simulink model "Chua_TxRx"  (R2020a)
settings: Solver=VariableStepAuto  StartTime=0.0  StopTime=140  RelTol=1e-3
values from neighbouring files (symbols this model uses):
  beta = -36    [SetupConstants.m]
  delay = 10    [SetupConstants.m]
  freq = 1/10    (= 0.1)    [SetupConstants.m]
libraries: simulink x1
settings Model: PacingRate=1.100000  Creator=RaviM  LastModifiedBy=RaviM

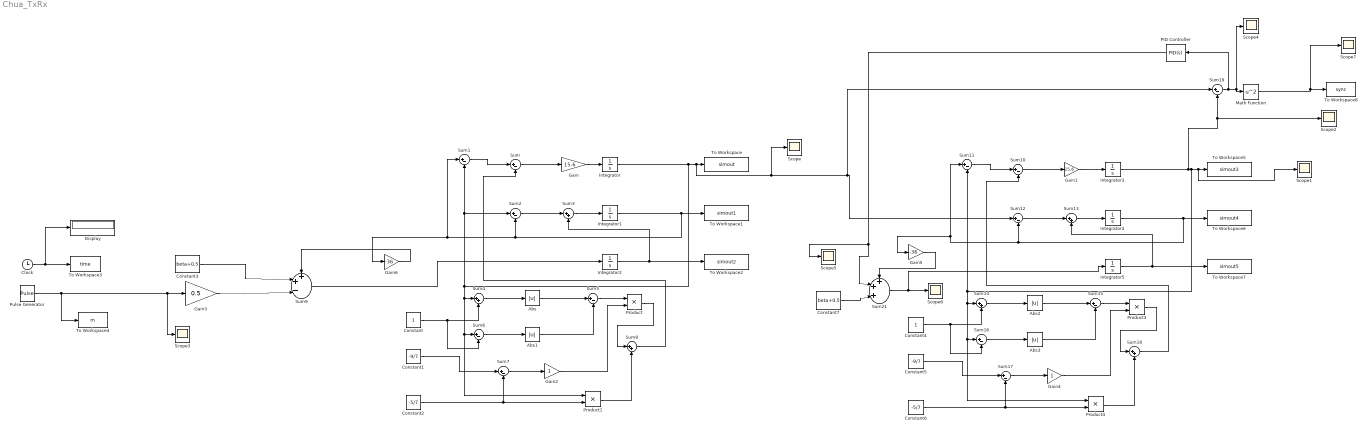
== system Chua_TxRx ==
  Abs{,1..3} (4 alike) : Abs
  Clock : Clock
  Constant : Constant
  Constant1 : Constant  Value=-9/7
  Constant2 : Constant  Value=-5/7
  Constant3 : Constant  Value=beta+0.5
  Constant4 : Constant
  Constant5 : Constant  Value=-9/7
  Constant6 : Constant  Value=-5/7
  Constant7 : Constant  Value=beta+0.5
  Display : Display
      settings: Decimation=5
  Gain : Gain  Gain=15.6
  Gain1 : Gain  Gain=15.6
  Gain2 : Gain
  Gain3 : Gain  Gain=0.5
  Gain4 : Gain
  Gain5 : Gain  Gain=-36
  Gain6 : Gain  Gain=-36
  Integrator{,1..5} (6 alike) : Integrator  InitialCondition=0.1
  Math Function : Math  Operator=square  SignedPower=on  SaturateOnIntegerOverflow=on
  PID Controller : simulink/Continuous/PID Controller  Controller=PID  Form=Ideal  TimeDomain=Continuous-time  UseExternalTs=off  SampleTime=-1  IntegratorMethod=Forward Euler  FilterMethod=Forward Euler  ControllerParametersSource=internal  P=.5  I=0.2  D=.0000004  UseFilter=on  N=100  TunerSelectOption=Transfer Function Based (PID Tuner App)  InitialConditionSource=internal  InitialConditionForIntegrator=0  InitialConditionForFilter=0  DifferentiatorICPrevScaledInput=0  ExternalReset=none  TrackingMode=off  Kt=1  LimitOutput=off  UpperSaturationLimit=inf  LowerSaturationLimit=-inf  LinearizeAsGain=on  AntiWindupMode=none  Kb=1  POutMin=[]  POutMax=[]  IOutMin=[]  IOutMax=[]  DOutMin=[]  DOutMax=[]  NOutMin=[]  NOutMax=[]  SumOutMin=[]  SumOutMax=[]  SaturationOutMin=[]  SaturationOutMax=[]  PParamMin=[]  PParamMax=[]  IParamMin=[]  IParamMax=[]  DParamMin=[]  DParamMax=[]  NParamMin=[]  NParamMax=[]  KbParamMin=[]  KbParamMax=[]  KtParamMin=[]  KtParamMax=[]  KbOutMin=[]  KbOutMax=[]  KtOutMin=[]  KtOutMax=[]  IntegratorOutMin=[]  IntegratorOutMax=[]  FilterOutMin=[]  FilterOutMax=[]  SumI1OutMin=[]  SumI1OutMax=[]  SumI2OutMin=[]  SumI2OutMax=[]  SumI3OutMin=[]  SumI3OutMax=[]  SumI4OutMin=[]  SumI4OutMax=[]  SumDOutMin=[]  SumDOutMax=[]  DifferentiatorOutMin=[]  DifferentiatorOutMax=[]  FilterDiffOutCoefMin=[]  FilterDiffOutCoefMax=[]  ReciprocalOutMin=[]  ReciprocalOutMax=[]  SumDenOutMin=[]  SumDenOutMax=[]  SumNumOutMin=[]  SumNumOutMax=[]  DivideOutMin=[]  DivideOutMax=[]  UdiffTsProdOutMin=[]  UdiffTsProdOutMax=[]  NTsProdOutMin=[]  NTsProdOutMax=[]  UintegralTsProdOutMin=[]  UintegralTsProdOutMax=[]  UngainTsProdOutMin=[]  UngainTsProdOutMax=[]  IntegratorContinuousStateAttributes=''  IntegratorStateMustResolveToSignalObject=off  IntegratorRTWStateStorageClass=Auto  FilterContinuousStateAttributes=''  FilterStateMustResolveToSignalObject=off  FilterRTWStateStorageClass=Auto  ParallelPVariant=Passthrough  IdealPVariant=InternalParameters  IVariant=InternalParameters  DVariant=InternalParameters  IntegratorVariant=Continuous  SatVariant=Disabled  AWVariant=Passthrough  PCopyVariant=Disabled  TRVariant=Disabled  FdbkBlocksVariant=Forward  IdealPFdbkVariant=Disabled  SatFdbkVariant=Disabled  DerivativeFilterVariant=ContFilter  NVariant=InternalParameters  NCopyVariant=Disabled  FilterICVariant=InternalICsFilter  IntegratorICVariant=InternalICs  ExternalResetVariant=Disabled  TRSumVariant=Passthrough  SumFdbkVariant=Disabled  SumVariant=Sum_PID  TsampFilterVariant=InternalTs  TsampNgainVariant=Passthrough  TsampIntegralVariant=Passthrough
  Product{,1,3..4} (4 alike) : Product
  Pulse Generator : DiscretePulseGenerator  PulseType=Time based  Period=2/freq  PulseWidth=50  PhaseDelay=delay
  Scope{,1..7} (8 alike) : Scope
  Sum{,1..2,5..7,10..12,15..17,19} (13 alike) : Sum  Inputs=|+-
  Sum{3..4,8,13..14,18} (6 alike) : Sum  Inputs=|++
  Sum21 : Sum  Inputs=+++|
  Sum9 : Sum  Inputs=++-|
  To Workspace : ToWorkspace  VariableName=simout  SaveFormat=Timeseries  SampleTime=-1
  To Workspace1 : ToWorkspace  VariableName=simout1  SaveFormat=Timeseries  SampleTime=-1
  To Workspace2 : ToWorkspace  VariableName=simout2  SaveFormat=Timeseries  SampleTime=-1
  To Workspace3 : ToWorkspace  VariableName=time  SampleTime=-1
  To Workspace4 : ToWorkspace  VariableName=m  SampleTime=-1
  To Workspace5 : ToWorkspace  VariableName=simout3  SaveFormat=Timeseries  SampleTime=-1
  To Workspace6 : ToWorkspace  VariableName=simout4  SaveFormat=Timeseries  SampleTime=-1
  To Workspace7 : ToWorkspace  VariableName=simout5  SaveFormat=Timeseries  SampleTime=-1
  To Workspace8 : ToWorkspace  VariableName=sync  SampleTime=-1
  wires:
  Constant2/1 -> Sum7/2, Product1/2
  Constant1/1 -> Sum7/1
  Sum7/1 -> Gain2/1
  Gain2/1 -> Product/2
  Product1/1 -> Sum8/2
  Product/1 -> Sum8/1
  Sum6/1 -> Abs1/1
  Sum4/1 -> Abs/1
  Abs/1 -> Sum5/1
  Abs1/1 -> Sum5/2
  Constant/1 -> Sum4/2, Sum6/2
  Sum8/1 -> Sum/2
  Sum1/1 -> Sum/1
  Sum/1 -> Gain/1
  Gain/1 -> Integrator/1
  Sum3/1 -> Integrator1/1
  Sum2/1 -> Sum3/1
  Integrator1/1 -> Gain6/1, Sum1/1, Sum2/2, To Workspace1/1
  Integrator2/1 -> To Workspace2/1, Sum3/2
  Gain6/1 -> Sum9/1
  Sum5/1 -> Product/1
  Gain3/1 -> Sum9/3
  Pulse Generator/1 -> To Workspace4/1, Scope3/1, Gain3/1
  Sum9/1 -> Integrator2/1
  Clock/1 -> Display/1, To Workspace3/1
  Constant3/1 -> Sum9/2
  Sum21/1 -> Integrator5/1, Scope6/1
  Gain5/1 -> Sum21/1
  Sum16/1 -> Abs3/1
  Sum17/1 -> Gain4/1
  Sum18/1 -> Sum10/2
  Constant6/1 -> Sum17/2, Product4/2
  Product3/1 -> Sum18/1
  Sum10/1 -> Gain1/1
  Gain4/1 -> Product3/2
  Product4/1 -> Sum18/2
  Gain1/1 -> Integrator3/1
  Sum11/1 -> Sum10/1
  Constant5/1 -> Sum17/1
  Sum12/1 -> Sum13/1
  Sum15/1 -> Product3/1
  Sum14/1 -> Abs2/1
  Sum13/1 -> Integrator4/1
  Abs3/1 -> Sum15/2
  Abs2/1 -> Sum15/1
  Constant4/1 -> Sum14/2, Sum16/2
  Integrator5/1 -> To Workspace7/1, Sum13/2
  Integrator4/1 -> Sum11/1, Gain5/1, Sum12/2, To Workspace6/1
  PID Controller/1 -> Sum21/2, Scope5/1
  Math Function/1 -> Scope7/1, To Workspace8/1
  Sum19/1 -> PID Controller/1, Scope4/1, Math Function/1
  Integrator/1 -> Sum2/1, Sum1/2, Product1/1, Sum6/1, Sum4/1, Sum19/1, Sum12/1, Scope/1, To Workspace/1
  Constant7/1 -> Sum21/3
  Integrator3/1 -> Scope2/1, Sum19/2, Sum11/2, Product4/1, Sum16/1, Sum14/1, Scope1/1, To Workspace5/1
